simulink model "unicycle_simple"  (R2021a)
settings: Solver=VariableStepAuto  StartTime=0.0  StopTime=10.0  MaxStep=1e-3  RelTol=1e-3
libraries: simulink x2
settings Model: EnablePacing=on  Creator=kjartan  LastModifiedBy=kjartan

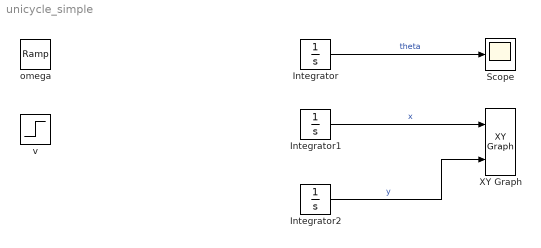
== system unicycle_simple ==
  Integrator : Integrator
  Integrator1 : Integrator
  Integrator2 : Integrator
  Scope : Scope
  XY Graph : simulink/Sinks/XY Graph  xmin=-2  xmax=2  ymin=-2  ymax=2  st=-1
  omega : simulink/Sources/Ramp  slope=1  start=0  InitialOutput=0
  v : Step  SampleTime=0
  wires:
  Integrator2/1 -> XY Graph/2  "y"
  Integrator1/1 -> XY Graph/1  "x"
  Integrator/1 -> Scope/1  "theta"
